simulink model "DFT"  (R2013a)
settings: Solver=ode45  StartTime=0.0  StopTime=2.0  RelTol=1e-3
libraries: powerlib_extras x4, dsparch4 x3
settings Model: Creator=NIT  LastModifiedBy=verma_sss
settings DataIOCC: SignalLoggingSaveFormat=ModelDataLogs
settings OptimizationCC: ExpressionDepthLimit=2147483647
settings DebuggingCC: FcnCallInpInsideContextMsg=UseLocalSettings
settings GRTTargetCC: CombineOutputUpdateFcns=off  GRTInterface=on

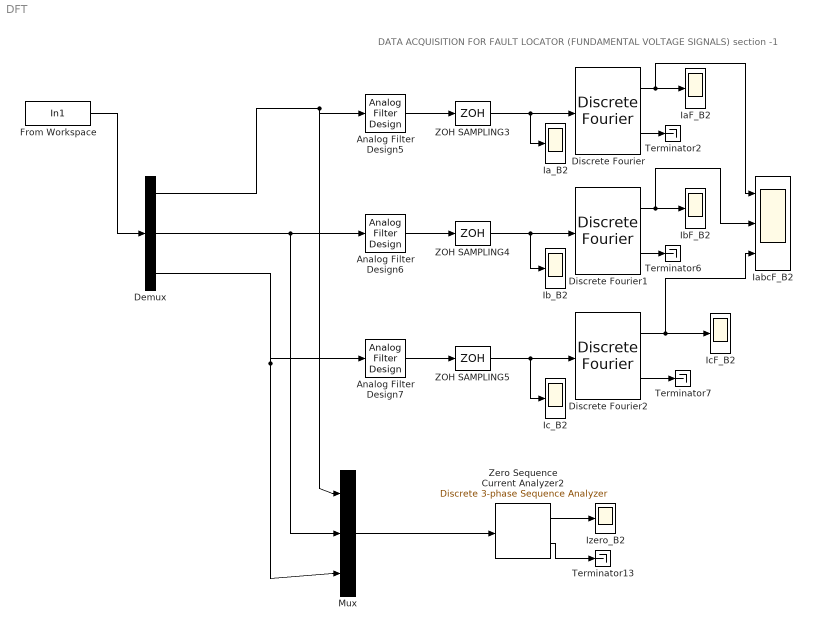
== system DFT ==
  note: DATA ACQUISITION FOR FAULT LOCATOR
      | (FUNDAMENTAL VOLTAGE SIGNALS) section -1
  " Izero_B2" : Scope
      settings: TimeRange=0.2  YMin=-1.5  YMax=1.5  SaveName=Izero_B2  MaxDataPoints=2001  SampleInput=on  SampleTime=1e-3
  Analog Filter Design5 : dsparch4/Analog Filter Design  method=Butterworth  filttype=Lowpass  N=2  Wlo=2*pi*400  Whi=80  Rp=2  Rs=40
  Analog Filter Design6 : dsparch4/Analog Filter Design  method=Butterworth  filttype=Lowpass  N=2  Wlo=2*pi*400  Whi=80  Rp=2  Rs=40
  Analog Filter Design7 : dsparch4/Analog Filter Design  method=Butterworth  filttype=Lowpass  N=2  Wlo=2*pi*400  Whi=80  Rp=2  Rs=40
  Demux : Demux  Outputs=3
  Discrete Fourier : powerlib_extras/Discrete Measurements/Discrete  Fourier  Freq=50  n=1  Par_Init=[0 0]  Ts=1e-3
  Discrete Fourier1 : powerlib_extras/Discrete Measurements/Discrete  Fourier  Freq=50  n=1  Par_Init=[0 0]  Ts=1e-3
  Discrete Fourier2 : powerlib_extras/Discrete Measurements/Discrete  Fourier  Freq=50  n=1  Par_Init=[0 0]  Ts=1e-3
  From Workspace : FromWorkspace  VariableName=In1  SampleTime=1e-3
  IaF_B2 : Scope
      settings: TimeRange=0.1  YMin=0  YMax=3000  SaveName=IaF_B2  MaxDataPoints=2000  SampleInput=on  SampleTime=1e-3
  Ia_B2 : Scope
      settings: TimeRange=0.2  YMin=-200000  YMax=200000  SaveName=Ia_B2  MaxDataPoints=2000  SampleInput=on  SampleTime=1e-3
  IabcF_B2 : Scope  NumInputPorts=3
      settings: TimeRange=1  YMin=-200000~-5~-5  YMax=200000~5~5  SaveName=Iabcf_B2  DataFormat=Structure  MaxDataPoints=2000  SampleInput=on  SampleTime=1e-3
  IbF_B2 : Scope
      settings: TimeRange=1  YMin=-200000  YMax=200000  SaveName=IbF_B2  MaxDataPoints=2000  SampleInput=on  SampleTime=1e-3
  Ib_B2 : Scope
      settings: TimeRange=0.2  YMin=-200000  YMax=200000  SaveName=Ib_B2  MaxDataPoints=2000  SampleInput=on  SampleTime=1e-3
  IcF_B2 : Scope
      settings: TimeRange=1  YMin=-200000  YMax=200000  SaveName=IcF_B2  MaxDataPoints=2000  SampleInput=on  SampleTime=1e-3
  Ic_B2 : Scope
      settings: TimeRange=0.2  YMin=-200000  YMax=200000  SaveName=Ic_B2  MaxDataPoints=2000  SampleInput=on  SampleTime=1e-3
  Mux : Mux  Inputs=3
  Terminator{2,6..7,13} (4 alike) : Terminator
  ZOH SAMPLING3 : ZeroOrderHold  SampleTime=1e-3
  ZOH SAMPLING4 : ZeroOrderHold  SampleTime=1e-3
  ZOH SAMPLING5 : ZeroOrderHold  SampleTime=1e-3
  Zero Sequence Current Analyzer2 : powerlib_extras/Discrete Measurements/Discrete 3-phase Sequence Analyzer  Freq=50  n=1  seq=Zero  Par_Init=[0 0]  Ts=1e-3
  wires:
  Discrete Fourier/1 -> IaF_B2/1, IabcF_B2/1
  Discrete Fourier1/1 -> IbF_B2/1, IabcF_B2/2
  Discrete Fourier2/1 -> IcF_B2/1, IabcF_B2/3
  Analog Filter Design5/1 -> ZOH SAMPLING3/1
  Analog Filter Design6/1 -> ZOH SAMPLING4/1
  Analog Filter Design7/1 -> ZOH SAMPLING5/1
  ZOH SAMPLING5/1 -> Ic_B2/1, Discrete Fourier2/1
  ZOH SAMPLING4/1 -> Ib_B2/1, Discrete Fourier1/1
  ZOH SAMPLING3/1 -> Discrete Fourier/1, Ia_B2/1
  Discrete Fourier/2 -> Terminator2/1
  Discrete Fourier1/2 -> Terminator6/1
  Discrete Fourier2/2 -> Terminator7/1
  Zero Sequence Current Analyzer2/1 -> " Izero_B2"/1
  Zero Sequence Current Analyzer2/2 -> Terminator13/1
  Demux/3 -> Analog Filter Design7/1, Mux/3
  Demux/2 -> Analog Filter Design6/1, Mux/2
  Mux/1 -> Zero Sequence Current Analyzer2/1
  Demux/1 -> Mux/1, Analog Filter Design5/1
  From Workspace/1 -> Demux/1
